simulink model "parte3_eje4_avr_exac2"  (R2017b)
settings: Solver=VariableStepAuto  StartTime=0.0  StopTime=10.0  RelTol=1e-3
values from neighbouring files (symbols this model uses):
  AEX = 0.014    [parte3_DC1A_data.m]    (also in parte3_eje3_EXAC1.m = 0.1; parte3_eje3_EXAC2.m = 0.1)
  BEX = 1.55    [parte3_DC1A_data.m]    (also in parte3_eje3_EXAC1.m = 0.03; parte3_eje3_EXAC2.m = 0.03)
  IFDfin = 1000    [parte3_eje3_EXAC1.m]    (also in parte3_eje3_EXAC2.m = 0; parte3_eje5_ESSTB.m = 1)
  Ka = 400    [parte3_eje3_EXAC1.m]    (also in parte3_eje3_EXAC2.m)
  KB = 100    [parte3_eje3_EXAC2.m]
  KC = 0.2    [parte3_eje3_EXAC1.m]    (also in parte3_eje3_EXAC2.m; parte3_eje5_ESSTB.m = 0.1; parte3_eje6_ESST1A.m = 0.01)
  KD = 0.38    [parte3_eje3_EXAC1.m]    (also in parte3_eje3_EXAC2.m)
  Ke = 1    [parte3_eje3_EXAC1.m]    (also in parte3_eje3_EXAC2.m)
  Kf = 0.03    [parte3_eje3_EXAC1.m]    (also in parte3_eje3_EXAC2.m)
  KH = 1    [parte3_eje3_EXAC2.m]
  KL = 1    [parte3_eje3_EXAC2.m]
  Ta = 0.02    [parte3_eje3_EXAC1.m]    (also in parte3_eje3_EXAC2.m; parte3_eje5_ESSTB.m = 0.01)
  Tb = 2    [parte3_eje3_EXAC1.m]    (also in parte3_eje3_EXAC2.m)
  Tc = 2    [parte3_eje3_EXAC1.m]    (also in parte3_eje3_EXAC2.m)
  Te = 0.8    [parte3_eje3_EXAC1.m]    (also in parte3_eje3_EXAC2.m)
  Tf = 1    [parte3_eje3_EXAC1.m]    (also in parte3_eje3_EXAC2.m)
  Tr = 0.01    [parte3_eje2_SMIB_Exc_graph.m]    (also in parte3_eje3_EXAC1.m; parte3_eje3_EXAC2.m; parte3_eje5_ESSTB.m = 0.3)
  Vrefin = 1    [parte3_eje3_EXAC1.m]    (also in parte3_eje3_EXAC2.m; parte3_eje5_ESSTB.m = 0.01)
  Vrmax = 15    [parte3_eje3_EXAC1.m]    (also in parte3_eje3_EXAC2.m)
  Vrmin = -15    [parte3_eje3_EXAC1.m]    (also in parte3_eje3_EXAC2.m)
settings Model: Creator=cjuar  LastModifiedBy=cjuar

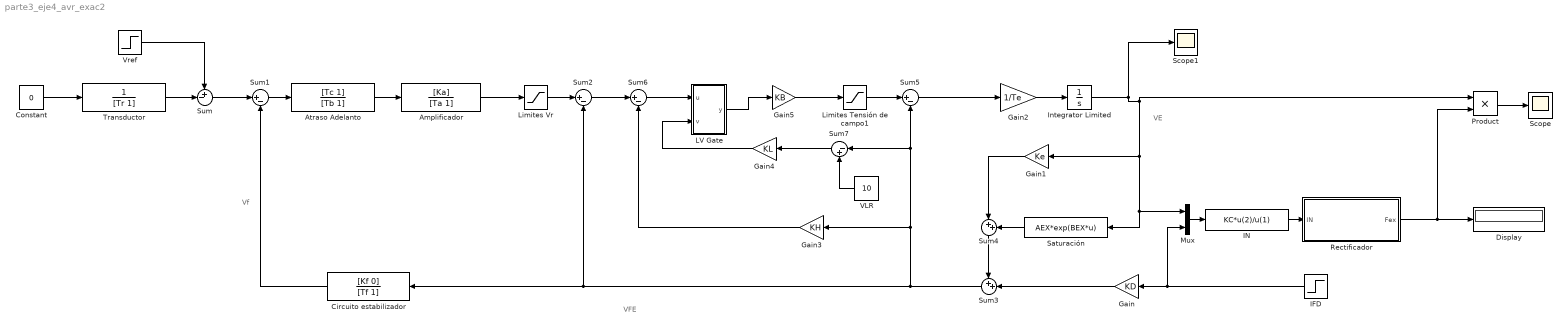
== system parte3_eje4_avr_exac2 ==
  note: Vf
  note: VFE
  note: VE
  Amplificador : TransferFcn  Numerator=[Ka]  Denominator=[Ta 1]
  Atraso Adelanto : TransferFcn  Numerator=[Tc 1]  Denominator=[Tb 1]
  Circuito estabilizador : TransferFcn  Numerator=[Kf 0]  Denominator=[Tf 1]
  Constant : Constant  Value=0
  Display : Display
  Gain : Gain  Gain=KD
  Gain1 : Gain  Gain=Ke
  Gain2 : Gain  Gain=1/Te
  Gain3 : Gain  Gain=KH
  Gain4 : Gain  Gain=KL
  Gain5 : Gain  Gain=KB
  IFD : Step  After=IFDfin  SampleTime=0
  IN : Fcn  Expr=KC*u(2)/u(1)
  Integrator Limited : Integrator  LimitOutput=on  UpperSaturationLimit=100  LowerSaturationLimit=0
  LV Gate : Subsystem
  Limites Tensión de campo1 : Saturate  UpperLimit=Vrmax  LowerLimit=Vrmin
  Limites Vr : Saturate  UpperLimit=Vrmax  LowerLimit=Vrmin
  Mux : Mux  Inputs=2
  Product : Product
  Rectificador : MATLAB Function  TreatAsAtomicUnit=on
  Saturación : Fcn  Expr=AEX*exp(BEX*u)
  Scope : Scope
  Scope1 : Scope
  Sum : Sum  Inputs=+-|
  Sum{1..2,5..6} (4 alike) : Sum  Inputs=|+-
  Sum3 : Sum  Inputs=++|
  Sum4 : Sum  Inputs=|++
  Sum7 : Sum  Inputs=|-+
  Transductor : TransferFcn  Denominator=[Tr 1]
  VLR : Constant  Value=10
  Vref : Step  After=Vrefin  SampleTime=0
  wires:
  Atraso Adelanto/1 -> Amplificador/1
  Product/1 -> Scope/1
  Saturación/1 -> Sum4/2
  Sum4/1 -> Sum3/1
  Sum1/1 -> Atraso Adelanto/1
  Gain2/1 -> Integrator Limited/1
  Vref/1 -> Sum/1
  Circuito estabilizador/1 -> Sum1/2
  Rectificador/1(Fex) -> Product/2, Display/1
  IN/1 -> Rectificador/1(IN)
  Mux/1 -> IN/1
  Sum3/1 -> Sum7/1, Sum5/2, Gain3/1, Sum2/2, Circuito estabilizador/1
  IFD/1 -> Mux/2, Gain/1
  Gain/1 -> Sum3/2
  Limites Vr/1 -> Sum2/1
  Transductor/1 -> Sum/2
  Sum/1 -> Sum1/1
  Gain1/1 -> Sum4/1
  Amplificador/1 -> Limites Vr/1
  Integrator Limited/1 -> Product/1, Mux/1, Saturación/1, Gain1/1, Scope1/1
  Constant/1 -> Transductor/1
  Sum5/1 -> Gain2/1
  Sum2/1 -> Sum6/1
  Sum6/1 -> LV Gate/1(u)
  Gain3/1 -> Sum6/2
  Gain4/1 -> LV Gate/2(v)
  Sum7/1 -> Gain4/1
  LV Gate/1(y) -> Gain5/1
  Limites Tensión de campo1/1 -> Sum5/1
  Gain5/1 -> Limites Tensión de campo1/1
  VLR/1 -> Sum7/2

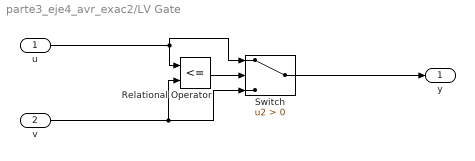
== system parte3_eje4_avr_exac2/LV Gate ==
  u : Inport
  v : Inport  Port=2
  Relational Operator : RelationalOperator  Operator=<=  OutDataTypeStr=boolean  RndMeth=Simplest
  Switch : Switch  Criteria=u2 > Threshold  InputSameDT=on
  y : Outport
  wires:
  u/1 -> Switch/1, Relational Operator/1
  Switch/1 -> y/1
  v/1 -> Switch/3, Relational Operator/2
  Relational Operator/1 -> Switch/2

== matlab function parte3_eje4_avr_exac2/Rectificador ==
  data: IN input; Fex output
function Fex = Rectificador(IN)
if IN<=0
    Fex=1;
elseif IN<=0.433
    Fex=1-0.577*IN;
elseif IN>0.433&&IN<0.75
    Fex=sqrt(0.75-IN^2);
elseif IN>=0.75&&IN<=1
    Fex=1.732*(1-IN);
else
    Fex=0;
end
